simulink model "TestStructure"  (R2022b)
settings: Solver=FixedStepDiscrete  StartTime=0.0  StopTime=300  FixedStep=SampleTime  RelTol=1e-3
InitFcn:
  | SampleTime = 0.001;
  | ButtonValue=0;
  | load("BusConfig.mat");
model workspace (MAT data in the model file):
  Manual_Auto = 1
  Pattern = 1
  Pause_Start = 1
  Stop = 1
  Unlock_Lock = 1
undefined symbols (not defined in the file or in its folder): DiscIntNeverNeededParam
libraries: dspfdesign x4, dspstat3 x4
(part 1 of 3)
settings Model: SimulationMode=external  ExtModeEnableFloating=off  ExplicitPartitioning=on  Creator=My-Dell-PC  LastModifiedBy=Lenovo
settings SolverCC: ConcurrentTasks=on  PositivePriorityOrder=on
settings OptimizationCC: BlockReduction=off  OptimizeBlockIOStorage=off
settings DebuggingCC: TasksWithSamePriorityMsg=none
settings HardwareCC: ProdBitPerLong=64  ProdLongLongMode=on  ProdHWDeviceType=Intel->x86-64 (Linux 64)
settings RTWCC: Description=Simulink Real-Time  SystemTargetFile=slrealtime.tlc  TemplateMakefile=slrealtime_default_tmf  Toolchain=Simulink Real-Time Toolchain  BuildConfiguration=Faster Runs  CodeExecutionProfiling=on  TargetLang=C++
settings CodeAppCC: MaxIdLength=128

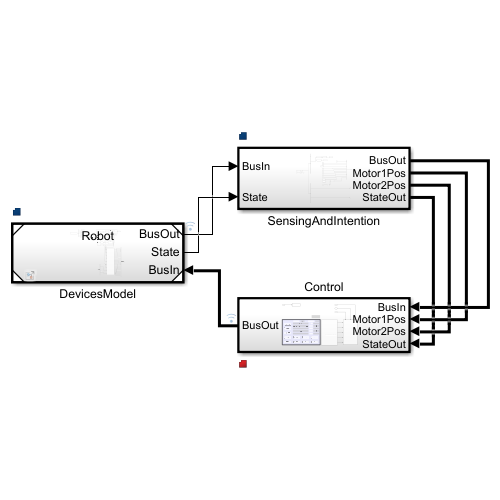
[thumbnail: Simulink's stored preview of the top-level diagram]
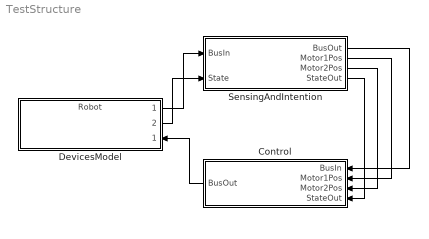
== system TestStructure ==
  Control : Subsystem  TreatAsAtomicUnit=on
  DevicesModel : ModelReference  ModelNameDialog=Robot.slx  SimulationMode=Normal  ModelReferenceVersion=1.102
      settings: PortSchema="{\"entries\":[{\"content\":{\"sides\":[{\"content\":{\"connectorIds\":[]},\"type\":\"ConnectorPlacement.EquallySpacedRectSide\",\"uuid\":\"7b8c9a1c-e183-4267-9de8-fd35f280369e\"},{\"content\":{\"connectorIds\":[\"Out1\",\"Out2\",\"In1\"],\"side\":\"RIGHT\"},\"type\":\"ConnectorPlacement.EquallySpacedRectSide\",\"uuid\":\"78ba3a26-fd01-47d1-83ec-a88a58443a5d\"},{\"content\":{\"connectorIds\":[],\"side\":\"TOP\"},\"type\":\"ConnectorPlacement.EquallySpacedRectSide\",\"uuid\":\"d4867a2f-46dd-4a62-ab42-9e8e97143c91\"}]},\"type\":\"ConnectorPlacement.EquallySpacedConnector\",\"uuid\":\"fb86ace7-67ae-423a-b56c-83b1d93efbca\"}],\"packageUris\":[\"http://schema.mathworks.com/mf0/Connector/R2020b\"],\"version\":\"1.0\"}"
  SensingAndIntention : Subsystem  TreatAsAtomicUnit=on
  wires:
  SensingAndIntention/1(BusOut) -> Control/1(BusIn)
  DevicesModel/1 -> SensingAndIntention/1(BusIn)
  Control/1(BusOut) -> DevicesModel/1
  SensingAndIntention/2(Motor1Pos) -> Control/2(Motor1Pos)
  SensingAndIntention/3(Motor2Pos) -> Control/3(Motor2Pos)
  DevicesModel/2 -> SensingAndIntention/2(State)
  SensingAndIntention/4(StateOut) -> Control/4(StateOut)

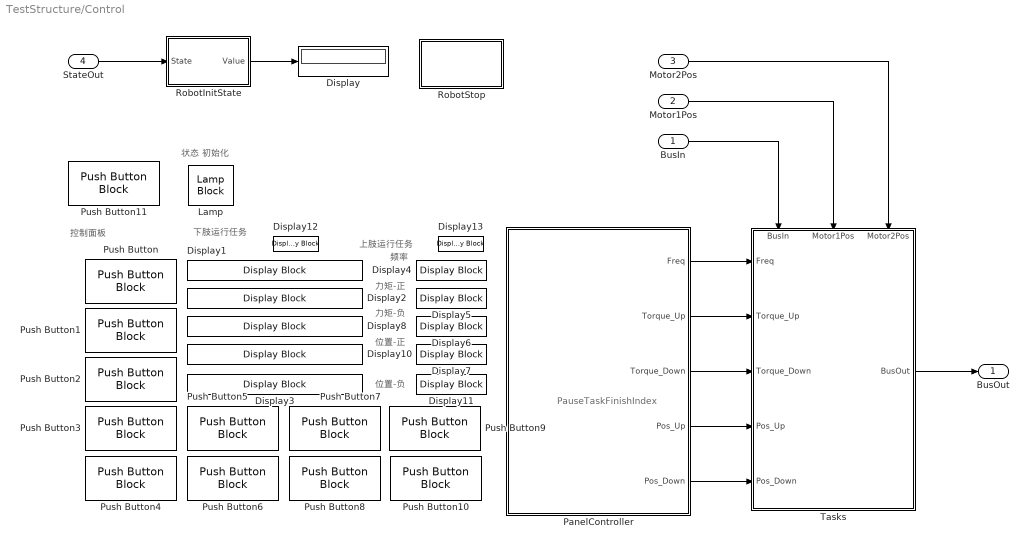
== system TestStructure/Control ==
  note: 状态 初始化
  note: PauseTaskFinishIndex
  note: 频率
  note: 控制面板
  note: 下肢运行任务
  note: 力矩-负
  note: 位置-负
  note: 位置-正
  note: 上肢运行任务
  note: 力矩-正
  BusIn : Inport  OutDataTypeStr=Bus: IntentionBus  BusOutputAsStruct=on
  Motor1Pos : Inport  Port=2
  Motor2Pos : Inport  Port=3
  StateOut : Inport  Port=4
  Display : Display
  Display{1..8,10..13} (12 alike) : DisplayBlock  LabelPosition=Hide  Transparency=1
  Lamp : LampBlock  LabelPosition=Hide
  PanelController : Subsystem  mask{LLFK_Freq_init=0.5, LLB_Freq_init=0.7, LLW_Freq_init=0.7, LLFK_Torque_Up_init=3, LLB_Torque_Up_init=9, LLW_Torque_Up_init=9, LLFK_Torque_Down_init=3, LLB_Torque_Down_init=9, LLW_Torque_Down_init=9, LLFK_Pos_Up_init=35, LLB_Pos_Up_init=80, LLW_Pos_Up_init=80, LLFK_Pos_Down_init=10, LLB_Pos_Down_init=120, LLW_Pos_Down_init=120}
      mask prompts: LLFK_Freq_init "LLFK_Freq_init (Hz)"; LLB_Freq_init "LLB_Freq_init (Hz)"; LLW_Freq_init "LLW_Freq_init (Hz)"; LLFK_Torque_Up_init "LLFK_Torque_Up_init (A)"; LLB_Torque_Up_init "LLB_Torque_Up_init (A)"; LLW_Torque_Up_init "LLW_Torque_Up_init (A)"; LLFK_Torque_Down_init "LLFK_Torque_Down_init (A)"; LLB_Torque_Down_init "LLB_Torque_Down_init (A)"; LLW_Torque_Down_init "LLW_Torque_Down_init (A)"; LLFK_Pos_Up_init "LLFK_Pos_Up_init (Degree)"; LLB_Pos_Up_init "LLB_Pos_Up_init (Degree)"; LLW_Pos_Up_init "LLW_Pos_Up_init (Degree)"; LLFK_Pos_Down_init "LLFK_Pos_Down_init (Degree)"; LLB_Pos_Down_init "LLB_Pos_Down_init (Degree)"; LLW_Pos_Down_init "LLW_Pos_Down_init (Degree)"
      mask DialogControl ParameterGroupVar Prompt: Freq_Init
      mask DialogControl Container3 Prompt: Torque_Up_Init
      mask DialogControl Container4 Prompt: Torque_Down_Init
      mask DialogControl Container5 Prompt: Pos_Up_init (Degree)
      mask DialogControl Container6 Prompt: Pos_Down_init (Degree)
  Push Button : PushButtonBlock  ButtonText=停止  Icon=Circle  IconColor=On  OffValue=0.000000
  Push Button1 : PushButtonBlock  ButtonText=启动/暂停  Icon=Circle  IconColor=On  OffValue=0.000000
  Push Button10 : PushButtonBlock  ButtonText=反方向-降  Icon=Circle  IconColor=On  OffValue=0.000000
  Push Button11 : PushButtonBlock  ButtonText=停止运行  Icon=Circle  IconColor=On  OffValue=0.000000
  Push Button2 : PushButtonBlock  ButtonText=模式  Icon=Circle  IconColor=On  OffValue=0.000000
  Push Button3 : PushButtonBlock  ButtonText=手动/自动  Icon=Circle  IconColor=On  OffValue=0.000000
  Push Button4 : PushButtonBlock  ButtonText=解锁/锁定  Icon=Circle  IconColor=On  OffValue=0.000000
  Push Button5 : PushButtonBlock  ButtonText=频率-升  Icon=Circle  IconColor=On  OffValue=0.000000
  Push Button6 : PushButtonBlock  ButtonText=频率-降  Icon=Circle  IconColor=On  OffValue=0.000000
  Push Button7 : PushButtonBlock  ButtonText=正方向-升  Icon=Circle  IconColor=On  OffValue=0.000000
  Push Button8 : PushButtonBlock  ButtonText=正方向-降  Icon=Circle  IconColor=On  OffValue=0.000000
  Push Button9 : PushButtonBlock  ButtonText=反方向-升  Icon=Circle  IconColor=On  OffValue=0.000000
  RobotInitState : Subsystem
  RobotStop : Subsystem
  Tasks : Subsystem
      settings: PortSchema="{\"entries\":[{\"content\":{\"sides\":[{\"content\":{\"connectorIds\":[\"In1\",\"In2\",\"In3\",\"In4\",\"In5\"]},\"type\":\"ConnectorPlacement.EquallySpacedRectSide\",\"uuid\":\"0ec11ac4-f889-444c-a7a1-b805f1cc982e\"},{\"content\":{\"connectorIds\":[\"Out1\"],\"side\":\"RIGHT\"},\"type\":\"ConnectorPlacement.EquallySpacedRectSide\",\"uuid\":\"b6409299-698f-49d2-9688-e152db4860ad\"},{\"content\":{\"connectorIds\":[\"In6\",\"In7\",\"In8\"],\"side\":\"TOP\"},\"type\":\"ConnectorPlacement.EquallySpacedRectSide\",\"uuid\":\"7591a67b-fad9-4669-8b21-584a47590ab5\"}]},\"type\":\"ConnectorPlacement.EquallySpacedConnector\",\"uuid\":\"b9f00c1f-80f2-4712-ac04-91dc0cbf24cb\"}],\"packageUris\":[\"http://schema.mathworks.com/mf0/Connector/R2020b\"],\"version\":\"1.0\"}"
  BusOut : Outport  OutDataTypeStr=Bus: ControlBus  BusOutputAsStruct=on
  wires:
  BusIn/1 -> Tasks/6(BusIn)
  PanelController/2(Torque_Up) -> Tasks/2(Torque_Up)
  PanelController/1(Freq) -> Tasks/1(Freq)
  PanelController/5(Pos_Down) -> Tasks/5(Pos_Down)
  PanelController/3(Torque_Down) -> Tasks/3(Torque_Down)
  PanelController/4(Pos_Up) -> Tasks/4(Pos_Up)
  Tasks/1(BusOut) -> BusOut/1
  Motor1Pos/1 -> Tasks/7(Motor1Pos)
  Motor2Pos/1 -> Tasks/8(Motor2Pos)
  StateOut/1 -> RobotInitState/1(State)
  RobotInitState/1(Value) -> Display/1

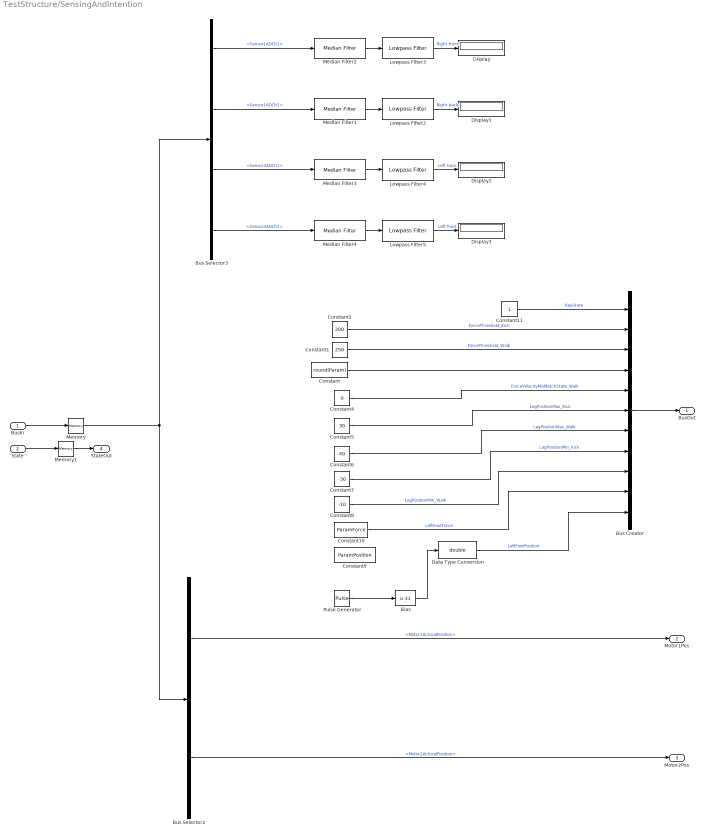
== system TestStructure/SensingAndIntention ==
  BusIn : Inport  OutDataTypeStr=Bus: SensingBus  BusOutputAsStruct=on
  State : Inport  Port=2
  Bias : Bias  Bias=-31  SaturateOnIntegerOverflow=off
  Bus Creator : BusCreator  Inputs=11  OutDataTypeStr=Bus: IntentionBus  NonVirtualBus=on
  Bus Selector2 : BusSelector  OutputSignals=Motor1ActuralPosition,Motor2ActuralPosition
  Bus Selector3 : BusSelector  OutputSignals=Sensor1ADCh1,Sensor1ADCh2,Sensor3ADCh1,Sensor3ADCh2
  Constant : Constant  Value=round(Param)  mask{Param=0.770}
  Constant1 : Constant  Value=250  OutDataTypeStr=double
  Constant10 : Constant  Value=ParamForce  OutDataTypeStr=double  mask{ParamForce=0.0}
  Constant11 : Constant  OutDataTypeStr=double
  Constant2 : Constant  Value=200  OutDataTypeStr=double
  Constant4 : Constant  Value=0  OutDataTypeStr=double
  Constant5 : Constant  Value=30  OutDataTypeStr=double
  Constant6 : Constant  Value=40  OutDataTypeStr=double
  Constant7 : Constant  Value=-30  OutDataTypeStr=double
  Constant8 : Constant  Value=-10  OutDataTypeStr=double
  Constant9 : Constant  Value=ParamPosition  OutDataTypeStr=double  mask{ParamPosition=1.860}
  Data Type Conversion : DataTypeConversion  OutDataTypeStr=double  SaturateOnIntegerOverflow=off  RndMeth=Floor
  Display{,1..3} (4 alike) : Display
  Lowpass Filter{2..5} (4 alike) : dspfdesign/Lowpass Filter  FilterType=IIR  DesignForMinimumOrder=off  FilterOrder=3  PassbandFrequency=3  StopbandFrequency=30  PassbandRipple=0.1  StopbandAttenuation=80  InheritSampleRate=off  SampleRate=1000  SimulateUsing=Code generation  roundingMode=Floor  coeffsDataTypeStr=fixdt(1,16)
  Median Filter{1..4} (4 alike) : dspstat3/Median Filter  WindowLength=80  SimulateUsing=Code generation
      settings: LibrarySourceBlock=|
      | dspfdesign/Median
      | Filter
  Memory : Memory
  Memory1 : Memory
  Pulse Generator : DiscretePulseGenerator  Amplitude=62  Period=T  PulseWidth=round(0.5*T)  PhaseDelay=round(0.5*T)  SampleTime=0.001  mask{T=2000.0}
  BusOut : Outport  OutDataTypeStr=Bus: IntentionBus  BusOutputAsStruct=on
  Motor1Pos : Outport  Port=2
  Motor2Pos : Outport  Port=3
  StateOut : Outport  Port=4
  wires:
  Bias/1 -> Data Type Conversion/1
  Constant1/1 -> Bus Creator/3  "ForceThreshold_Walk"
  Constant11/1 -> Bus Creator/1  "KeyState"
  Constant6/1 -> Bus Creator/7  "LegPositionMax_Walk"
  Data Type Conversion/1 -> Bus Creator/11  "LeftFootPosition"
  Constant2/1 -> Bus Creator/2  "ForceThreshold_Kick"
  Constant8/1 -> Bus Creator/9  "LegPositionMin_Walk"
  Constant7/1 -> Bus Creator/8  "LegPositionMin_Kick"
  Constant10/1 -> Bus Creator/10  "LeftFootForce"
  Constant4/1 -> Bus Creator/5  "ForceVelocityMisMatchState_Walk"
  Bus Creator/1 -> BusOut/1
  BusIn/1 -> Memory/1
  Constant5/1 -> Bus Creator/6  "LegPositionMax_Kick"
  Pulse Generator/1 -> Bias/1
  Bus Selector2/1 -> Motor1Pos/1  "<Motor1ActuralPosition>"
  Bus Selector2/2 -> Motor2Pos/1  "<Motor2ActuralPosition>"
  Memory/1 -> Bus Selector2/1, Bus Selector3/1
  Constant/1 -> Bus Creator/4
  Memory1/1 -> StateOut/1
  State/1 -> Memory1/1
  Median Filter1/1 -> Lowpass Filter2/1
  Median Filter2/1 -> Lowpass Filter3/1
  Bus Selector3/3 -> Median Filter3/1  "<Sensor3ADCh1>"
  Bus Selector3/1 -> Median Filter2/1  "<Sensor1ADCh1>"
  Median Filter4/1 -> Lowpass Filter5/1
  Bus Selector3/2 -> Median Filter1/1  "<Sensor1ADCh2>"
  Bus Selector3/4 -> Median Filter4/1  "<Sensor3ADCh2>"
  Median Filter3/1 -> Lowpass Filter4/1
  Lowpass Filter3/1 -> Display/1  "Right front"
  Lowpass Filter2/1 -> Display1/1  "Right back"
  Lowpass Filter4/1 -> Display2/1  "Left back"
  Lowpass Filter5/1 -> Display3/1  "Left front"

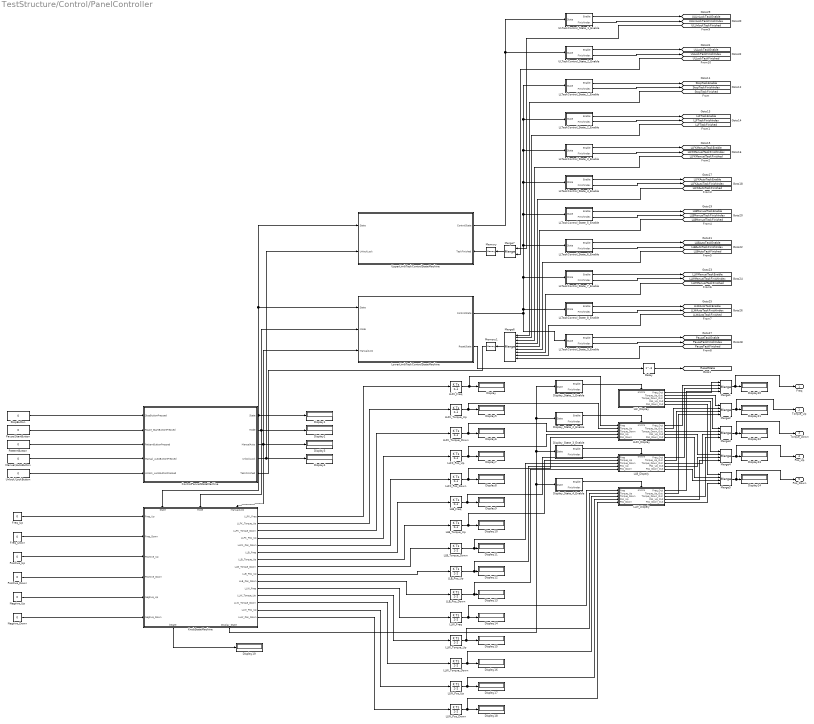
== system TestStructure/Control/PanelController ==
  ControlPannelStateMachine : Stateflow chart  TreatAsAtomicUnit=on
      settings: PortSchema="{\"entries\":[{\"content\":{\"sides\":[{\"content\":{\"connectorIds\":[\"In2\",\"In3\",\"In4\",\"In5\",\"In6\"]},\"type\":\"ConnectorPlacement.EquallySpacedRectSide\",\"uuid\":\"eab411cf-4b6a-48c6-b596-b66f8c420e7c\"},{\"content\":{\"connectorIds\":[\"Out1\",\"Out2\",\"Out3\",\"Out4\",\"In1\"],\"side\":\"RIGHT\"},\"type\":\"ConnectorPlacement.EquallySpacedRectSide\",\"uuid\":\"e0e09f46-7c1c-4140-8220-034119073277\"},{\"content\":{\"connectorIds\":[],\"side\":\"TOP\"},\"type\":\"ConnectorPlacement.EquallySpacedRectSide\",\"uuid\":\"ed6bf201-0ea3-4e7c-82a9-322f02ea728a\"}]},\"type\":\"ConnectorPlacement.EquallySpacedConnector\",\"uuid\":\"aa71b69e-402d-40b0-a3fd-c9400a9adadc\"}],\"packageUris\":[\"http://schema.mathworks.com/mf0/Connector/R2020b\"],\"version\":\"1.0\"}"
  Delay : Delay  DelayLength=3
  Display{,1..24} (25 alike) : Display
  Display_State_1_Enable : Subsystem  mask{TaskIndex=1}
  Display_State_2_Enable : Subsystem  mask{TaskIndex=2}
  Display_State_3_Enable : Subsystem  mask{TaskIndex=3}
  Display_State_4_Enable : Subsystem  mask{TaskIndex=4}
  Freq_Down : Constant  Value=0
  Freq_Up : Constant  Value=0
  KnobStateMachine : Stateflow chart  TreatAsAtomicUnit=on
      settings: PortSchema="{\"entries\":[{\"content\":{\"sides\":[{\"content\":{\"connectorIds\":[\"In1\",\"In2\",\"In3\",\"In4\",\"In5\",\"In6\"]},\"type\":\"ConnectorPlacement.EquallySpacedRectSide\",\"uuid\":\"78a56fe3-ceb0-42ee-90bc-aa39a12c9afb\"},{\"content\":{\"connectorIds\":[\"Out5\",\"Out3\",\"Out4\",\"Out6\",\"Out7\",\"Out8\",\"Out9\",\"Out10\",\"Out11\",\"Out12\",\"Out13\",\"Out14\",\"Out15\",\"Out16\",\"Out17\"],\"side\":\"RIGHT\"},\"type\":\"ConnectorPlacement.EquallySpacedRectSide\",\"uuid\":\"7553af84-a921-4f96-ace4-e42d4d568d32\"},{\"content\":{\"connectorIds\":[\"In7\",\"In8\",\"In9\"],\"side\":\"TOP\"},\"type\":\"ConnectorPlacement.EquallySpacedRectSide\",\"uuid\":\"299fd0e5-cc5b-4534-8b50-a134eaae2b47\"},{\"content\":{\"connectorIds\":[\"Out1\",\"Out2\"],\"side\":\"BOTTOM\"},\"type\":\"ConnectorPlacement.EquallySpacedRectSide\",\"uuid\":\"12262c62-fe5d-4494-9572-224afcc612c3\"}]},\"type\":\"ConnectorPlacement.EquallySpacedConnector\",\"uuid\":\"b0bd0f4e-3cef-462f-91f5-f8bdfcbb196f\"}],\"packageUris\":[\"http://schema.mathworks.com/mf0/Connector/R2020b\"],\"version\":\"1.0\"}"
  LLB_Dispaly : Subsystem
  LLB_Freq : DiscreteIntegrator  gainval=1000*0.1  InitialCondition=LLB_Freq_init  SampleTime=-1  LimitOutput=on  UpperSaturationLimit=2.5  LowerSaturationLimit=0.3  ICPrevOutput=DiscIntNeverNeededParam  ICPrevScaledInput=DiscIntNeverNeededParam
  LLB_Pos_Down : DiscreteIntegrator  gainval=1000*1  InitialCondition=LLB_Pos_Down_init  SampleTime=-1  LimitOutput=on  UpperSaturationLimit=140  LowerSaturationLimit=5  ICPrevOutput=DiscIntNeverNeededParam  ICPrevScaledInput=DiscIntNeverNeededParam
  LLB_Pos_Up : DiscreteIntegrator  gainval=1000*1  InitialCondition=LLB_Pos_Up_init  SampleTime=-1  LimitOutput=on  UpperSaturationLimit=100  LowerSaturationLimit=10  ICPrevOutput=DiscIntNeverNeededParam  ICPrevScaledInput=DiscIntNeverNeededParam
  LLB_Torque_Down : DiscreteIntegrator  gainval=1000*0.1  InitialCondition=LLB_Torque_Down_init  SampleTime=-1  LimitOutput=on  UpperSaturationLimit=10  LowerSaturationLimit=0  ICPrevOutput=DiscIntNeverNeededParam  ICPrevScaledInput=DiscIntNeverNeededParam
  LLB_Torque_Up : DiscreteIntegrator  gainval=1000*0.1  InitialCondition=LLB_Torque_Up_init  SampleTime=-1  LimitOutput=on  UpperSaturationLimit=10  LowerSaturationLimit=0  ICPrevOutput=DiscIntNeverNeededParam  ICPrevScaledInput=DiscIntNeverNeededParam
  LLFK_Display : Subsystem
  LLFK_Freq : DiscreteIntegrator  gainval=1000*0.1  InitialCondition=LLFK_Freq_init  SampleTime=-1  LimitOutput=on  UpperSaturationLimit=2.5  LowerSaturationLimit=0.3  ICPrevOutput=DiscIntNeverNeededParam  ICPrevScaledInput=DiscIntNeverNeededParam
  LLFK_Pos_Down : DiscreteIntegrator  gainval=1000*1  InitialCondition=LLFK_Pos_Down_init  SampleTime=-1  LimitOutput=on  UpperSaturationLimit=140  LowerSaturationLimit=5  ICPrevOutput=DiscIntNeverNeededParam  ICPrevScaledInput=DiscIntNeverNeededParam
  LLFK_Pos_Up : DiscreteIntegrator  gainval=1000*1  InitialCondition=LLFK_Pos_Up_init  SampleTime=-1  LimitOutput=on  UpperSaturationLimit=100  LowerSaturationLimit=10  ICPrevOutput=DiscIntNeverNeededParam  ICPrevScaledInput=DiscIntNeverNeededParam
  LLFK_Torque_Down : DiscreteIntegrator  gainval=1000*0.1  InitialCondition=LLFK_Torque_Down_init  SampleTime=-1  LimitOutput=on  UpperSaturationLimit=10  LowerSaturationLimit=0  ICPrevOutput=DiscIntNeverNeededParam  ICPrevScaledInput=DiscIntNeverNeededParam
  LLFK_Torque_Up : DiscreteIntegrator  gainval=1000*0.1  InitialCondition=LLFK_Torque_Up_init  SampleTime=-1  LimitOutput=on  UpperSaturationLimit=10  LowerSaturationLimit=0  ICPrevOutput=DiscIntNeverNeededParam  ICPrevScaledInput=DiscIntNeverNeededParam
  LLF_Display : Subsystem
  LLTaskControl_State_1_Enable : Subsystem  mask{TaskIndex=1}
  LLTaskControl_State_2_Enable : Subsystem  mask{TaskIndex=2}
  LLTaskControl_State_3_Enable : Subsystem  mask{TaskIndex=3}
  LLTaskControl_State_4_Enable : Subsystem  mask{TaskIndex=4}
  LLTaskControl_State_5_Enable : Subsystem  mask{TaskIndex=5}
  LLTaskControl_State_6_Enable : Subsystem  mask{TaskIndex=6}
  LLTaskControl_State_7_Enable : Subsystem  mask{TaskIndex=7}
  LLTaskControl_State_8_Enable : Subsystem  mask{TaskIndex=8}
  LLTaskControl_State_9_Enable : Subsystem  mask{TaskIndex=9}
  LLW_Dispaly : Subsystem
  LLW_Freq : DiscreteIntegrator  gainval=1000*0.1  InitialCondition=LLW_Freq_init  SampleTime=-1  LimitOutput=on  UpperSaturationLimit=2.5  LowerSaturationLimit=0.3  ICPrevOutput=DiscIntNeverNeededParam  ICPrevScaledInput=DiscIntNeverNeededParam
  LLW_Pos_Down : DiscreteIntegrator  gainval=1000*1  InitialCondition=LLW_Pos_Down_init  SampleTime=-1  LimitOutput=on  UpperSaturationLimit=140  LowerSaturationLimit=5  ICPrevOutput=DiscIntNeverNeededParam  ICPrevScaledInput=DiscIntNeverNeededParam
  LLW_Pos_Up : DiscreteIntegrator  gainval=1000*1  InitialCondition=LLW_Pos_Up_init  SampleTime=-1  LimitOutput=on  UpperSaturationLimit=100  LowerSaturationLimit=10  ICPrevOutput=DiscIntNeverNeededParam  ICPrevScaledInput=DiscIntNeverNeededParam
  LLW_Torque_Down : DiscreteIntegrator  gainval=1000*0.1  InitialCondition=LLW_Torque_Down_init  SampleTime=-1  LimitOutput=on  UpperSaturationLimit=10  LowerSaturationLimit=0  ICPrevOutput=DiscIntNeverNeededParam  ICPrevScaledInput=DiscIntNeverNeededParam
  LLW_Torque_Up : DiscreteIntegrator  gainval=1000*0.1  InitialCondition=LLW_Torque_Up_init  SampleTime=-1  LimitOutput=on  UpperSaturationLimit=10  LowerSaturationLimit=0  ICPrevOutput=DiscIntNeverNeededParam  ICPrevScaledInput=DiscIntNeverNeededParam
  LowerLimbTaskControlStateMachine : Stateflow chart  TreatAsAtomicUnit=on
  Manual/AutoButton : Constant  Value=0
  Memory : Memory
  Memory1 : Memory
  Merge{1..5} (5 alike) : Merge  Inputs=4
  Merge6 : Merge  Inputs=9
  Merge7 : Merge
  Negtive_Down : Constant  Value=0
  Negtive_Up : Constant  Value=0
  PatternButton : Constant  Value=0
  Pause/StartButton : Constant  Value=0
  Positive_Down : Constant  Value=0
  Positive_Up : Constant  Value=0
  StopButton : Constant  Value=0
  ULTaskControl_State_1_Enable : Subsystem  mask{TaskIndex=1}
  ULTaskControl_State_2_Enable : Subsystem  mask{TaskIndex=2}
  Unlock/LockButton : Constant  Value=0
  UpperLimbTaskControlStateMachine : Stateflow chart  TreatAsAtomicUnit=on
      settings: PortSchema="{\"entries\":[{\"content\":{\"sides\":[{\"content\":{\"connectorIds\":[\"In2\",\"In3\"]},\"type\":\"ConnectorPlacement.EquallySpacedRectSide\",\"uuid\":\"db13f0a7-324e-407f-8bcd-77b68e0b14b1\"},{\"content\":{\"connectorIds\":[\"Out1\",\"In1\"],\"side\":\"RIGHT\"},\"type\":\"ConnectorPlacement.EquallySpacedRectSide\",\"uuid\":\"09ee7819-fd71-4fe3-966c-1072161e5215\"},{\"content\":{\"connectorIds\":[],\"side\":\"TOP\"},\"type\":\"ConnectorPlacement.EquallySpacedRectSide\",\"uuid\":\"7aa19da4-9a31-402b-a0a8-4c1e281f7350\"}]},\"type\":\"ConnectorPlacement.EquallySpacedConnector\",\"uuid\":\"341b49cf-d13f-4e39-8c92-8137a597871d\"}],\"packageUris\":[\"http://schema.mathworks.com/mf0/Connector/R2020b\"],\"version\":\"1.0\"}"
  Freq : Outport
  Torque_Up : Outport  Port=2
  Torque_Down : Outport  Port=3
  Pos_Up : Outport  Port=4
  Pos_Down : Outport  Port=5
  tag scope: LLBAutoTaskEnable=global, LLBAutoTaskFinishIndex=global, LLBManualTaskEnable=global, LLBManualTaskFinishIndex=global, LLFKAutoTaskEnable=global, LLFKAutoTaskFinishIndex=global, LLFKManualTaskEnable=global, LLFKManualTaskFinishIndex=global, LLFTaskEnable=global, LLFTaskFinishIndex=global, LLWAutoTaskEnable=global, LLWAutoTaskFinishIndex=global, LLWManualTaskEnable=global, LLWManualTaskFinishIndex=global, PauseTaskEnable=global, PauseTaskFinishIndex=global, ResetState=global, StopTaskEnable=global, StopTaskFinishIndex=global, ULLockTaskEnable=global, ULLockTaskFinishIndex=global, ULUnLockTaskEnable=global, ULUnLockTaskFinishIndex=global
  wires:
  StopButton/1 -> ControlPannelStateMachine/2(StopButtonPressed)
  ControlPannelStateMachine/1(State) -> UpperLimbTaskControlStateMachine/2(State), LowerLimbTaskControlStateMachine/1(State), Display1/1, KnobStateMachine/7(State)
  Pause/StartButton/1 -> ControlPannelStateMachine/3(Pause_StartButtonPressed)
  PatternButton/1 -> ControlPannelStateMachine/4(PatternButtonPressed)
  Manual/AutoButton/1 -> ControlPannelStateMachine/5(Manual_AutoButtonPressed)
  ControlPannelStateMachine/2(Mode) -> KnobStateMachine/8(Mode), Display2/1, LowerLimbTaskControlStateMachine/2(Mode)
  ControlPannelStateMachine/3(ManualAuto) -> KnobStateMachine/9(ManualAuto), Display3/1, LowerLimbTaskControlStateMachine/3(ManualAuto)
  Unlock/LockButton/1 -> ControlPannelStateMachine/6(Unlock_LockButtonPressed)
  ControlPannelStateMachine/4(UnlockLock) -> Display4/1, UpperLimbTaskControlStateMachine/3(UnlockLock)
  LLFK_Freq/1 -> LLFK_Display/1(Freq), Display/1
  LLFK_Pos_Down/1 -> LLFK_Display/5(Pos_Down), Display8/1
  LLFK_Pos_Up/1 -> LLFK_Display/4(Pos_Up), Display7/1
  LLFK_Torque_Down/1 -> LLFK_Display/3(Torque_Down), Display6/1
  LLFK_Torque_Up/1 -> LLFK_Display/2(Torque_Up), Display5/1
  KnobStateMachine/5(LLFK_Freq) -> LLFK_Freq/1
  KnobStateMachine/3(LLFK_Torque_Up) -> LLFK_Torque_Up/1
  KnobStateMachine/4(LLFK_Torque_Down) -> LLFK_Torque_Down/1
  KnobStateMachine/6(LLFK_Pos_Up) -> LLFK_Pos_Up/1
  KnobStateMachine/7(LLFK_Pos_Down) -> LLFK_Pos_Down/1
  Freq_Up/1 -> KnobStateMachine/1(Freq_Up)
  Freq_Down/1 -> KnobStateMachine/2(Freq_Down)
  Positive_Up/1 -> KnobStateMachine/3(Positive_Up)
  Positive_Down/1 -> KnobStateMachine/4(Positive_Down)
  Negtive_Up/1 -> KnobStateMachine/5(Negtive_Up)
  Negtive_Down/1 -> KnobStateMachine/6(Negtive_Down)
  KnobStateMachine/9(LLB_Torque_Up) -> LLB_Torque_Up/1
  LLB_Pos_Up/1 -> LLB_Dispaly/4(Pos_Up), Display12/1
  KnobStateMachine/11(LLB_Pos_Up) -> LLB_Pos_Up/1
  LLB_Torque_Down/1 -> Display11/1, LLB_Dispaly/3(Torque_Down)
  LLB_Pos_Down/1 -> LLB_Dispaly/5(Pos_Down), Display13/1
  KnobStateMachine/10(LLB_Torque_Down) -> LLB_Torque_Down/1
  KnobStateMachine/12(LLB_Pos_Down) -> LLB_Pos_Down/1
  LLB_Freq/1 -> LLB_Dispaly/1(Freq), Display9/1
  LLB_Torque_Up/1 -> Display10/1, LLB_Dispaly/2(Torque_Up)
  KnobStateMachine/8(LLB_Freq) -> LLB_Freq/1
  KnobStateMachine/14(LLW_Torque_Up) -> LLW_Torque_Up/1
  LLW_Pos_Up/1 -> LLW_Dispaly/4(Pos_Up), Display17/1
  KnobStateMachine/16(LLW_Pos_Up) -> LLW_Pos_Up/1
  LLW_Torque_Down/1 -> LLW_Dispaly/3(Torque_Down), Display16/1
  KnobStateMachine/15(LLW_Torque_Down) -> LLW_Torque_Down/1
  KnobStateMachine/17(LLW_Pos_Down) -> LLW_Pos_Down/1
  LLW_Freq/1 -> LLW_Dispaly/1(Freq), Display14/1
  KnobStateMachine/13(LLW_Freq) -> LLW_Freq/1
  LLW_Torque_Up/1 -> LLW_Dispaly/2(Torque_Up), Display15/1
  LLW_Pos_Down/1 -> LLW_Dispaly/5(Pos_Down), Display18/1
  KnobStateMachine/1(kState) -> Display19/1
  Display_State_1_Enable/1(Enable) -> LLF_Display/Enable
  Display_State_2_Enable/1(Enable) -> LLFK_Display/Enable
  Display_State_3_Enable/1(Enable) -> LLB_Dispaly/Enable
  Display_State_4_Enable/1(Enable) -> LLW_Dispaly/Enable
  Merge1/1 -> Freq/1, Display20/1
  Merge2/1 -> Torque_Up/1, Display21/1
  Merge3/1 -> Torque_Down/1, Display22/1
  Merge4/1 -> Pos_Up/1, Display23/1
  Merge5/1 -> Pos_Down/1, Display24/1
  KnobStateMachine/2(Display_State) -> Display_State_1_Enable/1(State), Display_State_2_Enable/1(State), Display_State_3_Enable/1(State), Display_State_4_Enable/1(State)
  LLF_Display/1(Freq_Out) -> Merge1/1
  LLFK_Display/1(Freq_Out) -> Merge1/2
  LLB_Dispaly/1(Freq_Out) -> Merge1/3
  LLW_Dispaly/1(Freq_Out) -> Merge1/4
  LLF_Display/2(Torque_Up_Out) -> Merge2/1
  LLFK_Display/2(Torque_Up_Out) -> Merge2/2
  LLB_Dispaly/2(Torque_Up_Out) -> Merge2/3
  LLW_Dispaly/2(Torque_Up_Out) -> Merge2/4
  LLF_Display/3(Torque_Down_Out) -> Merge3/1
  LLFK_Display/3(Torque_Down_Out) -> Merge3/2
  LLB_Dispaly/3(Torque_Down_Out) -> Merge3/3
  LLW_Dispaly/3(Torque_Down_Out) -> Merge3/4
  LLF_Display/4(Pos_Up_Out) -> Merge4/1
  LLFK_Display/4(Pos_Up_Out) -> Merge4/2
  LLB_Dispaly/4(Pos_Up_Out) -> Merge4/3
  LLW_Dispaly/4(Pos_Up_Out) -> Merge4/4
  LLF_Display/5(Pos_Down_Out) -> Merge5/1
  LLFK_Display/5(Pos_Down_Out) -> Merge5/2
  LLB_Dispaly/5(Pos_Down_Out) -> Merge5/3
  LLW_Dispaly/5(Pos_Down_Out) -> Merge5/4
  [StopTaskFinished] -> Merge6/1
  LowerLimbTaskControlStateMachine/1(ControlState) -> LLTaskControl_State_1_Enable/1(State), LLTaskControl_State_2_Enable/1(State), LLTaskControl_State_3_Enable/1(State), LLTaskControl_State_4_Enable/1(State), LLTaskControl_State_5_Enable/1(State), LLTaskControl_State_6_Enable/1(State), LLTaskControl_State_7_Enable/1(State), LLTaskControl_State_8_Enable/1(State), LLTaskControl_State_9_Enable/1(State)
  Merge6/1 -> Memory1/1
  [LLFTaskFinished] -> Merge6/2
  [LLFKManualTaskFinished] -> Merge6/3
  [LLBManualTaskFinished] -> Merge6/5
  [LLWManualTaskFinished] -> Merge6/7
  [PauseTaskFinished] -> Merge6/9
  [LLFKAutoTaskFinished] -> Merge6/4
  [LLBAutoTaskFinished] -> Merge6/6
  [LLWAutoTaskFinished] -> Merge6/8
  Merge7/1 -> Memory/1
  [ULUnlockTaskFinished] -> Merge7/1
  [ULLockTaskFinished] -> Merge7/2
  UpperLimbTaskControlStateMachine/1(ControlState) -> ULTaskControl_State_2_Enable/1(State), ULTaskControl_State_1_Enable/1(State)
  LLTaskControl_State_8_Enable/1(Enable) -> [LLWAutoTaskEnable]
  LLTaskControl_State_5_Enable/2(FinishIndex) -> [LLBManualTaskFinishIndex]
  LLTaskControl_State_8_Enable/2(FinishIndex) -> [LLWAutoTaskFinishIndex]
  LLTaskControl_State_7_Enable/2(FinishIndex) -> [LLWManualTaskFinishIndex]
  LLTaskControl_State_1_Enable/2(FinishIndex) -> [StopTaskFinishIndex]
  LLTaskControl_State_3_Enable/1(Enable) -> [LLFKManualTaskEnable]
  ULTaskControl_State_2_Enable/1(Enable) -> [ULLockTaskEnable]
  LLTaskControl_State_4_Enable/1(Enable) -> [LLFKAutoTaskEnable]
  ULTaskControl_State_1_Enable/2(FinishIndex) -> [ULUnLockTaskFinishIndex]
  LLTaskControl_State_9_Enable/1(Enable) -> [PauseTaskEnable]
  LLTaskControl_State_9_Enable/2(FinishIndex) -> [PauseTaskFinishIndex]
  LLTaskControl_State_3_Enable/2(FinishIndex) -> [LLFKManualTaskFinishIndex]
  LLTaskControl_State_4_Enable/2(FinishIndex) -> [LLFKAutoTaskFinishIndex]
  LLTaskControl_State_5_Enable/1(Enable) -> [LLBManualTaskEnable]
  LLTaskControl_State_2_Enable/1(Enable) -> [LLFTaskEnable]
  LLTaskControl_State_2_Enable/2(FinishIndex) -> [LLFTaskFinishIndex]
  LLTaskControl_State_1_Enable/1(Enable) -> [StopTaskEnable]
  LLTaskControl_State_6_Enable/2(FinishIndex) -> [LLBAutoTaskFinishIndex]
  LLTaskControl_State_6_Enable/1(Enable) -> [LLBAutoTaskEnable]
  ULTaskControl_State_2_Enable/2(FinishIndex) -> [ULLockTaskFinishIndex]
  LLTaskControl_State_7_Enable/1(Enable) -> [LLWManualTaskEnable]
  ULTaskControl_State_1_Enable/1(Enable) -> [ULUnLockTaskEnable]
  Memory/1 -> UpperLimbTaskControlStateMachine/1(TaskFinished)
  Memory1/1 -> ControlPannelStateMachine/1(TaskFinished)
  Delay/1 -> [ResetState]
  LowerLimbTaskControlStateMachine/2(ResetState) -> Delay/1

== system TestStructure/Control/RobotInitState ==
  State : Inport
  Constant : Constant  Value=0
  Constant1 : Constant
  If : If  IfExpression=u1 == 5
  If Action Subsystem : Subsystem  TreatAsAtomicUnit=on
  If Action Subsystem1 : Subsystem  TreatAsAtomicUnit=on
  Merge1 : Merge
  Value : Outport
  wires:
  If Action Subsystem1/1(Out1) -> Merge1/2
  State/1 -> If/1
  If/1 -> If Action Subsystem/Action
  If Action Subsystem/1(Out1) -> Merge1/1
  Constant1/1 -> If Action Subsystem/1(In1)
  If/2 -> If Action Subsystem1/Action
  Constant/1 -> If Action Subsystem1/1(In1)
  Merge1/1 -> Value/1

== system TestStructure/Control/RobotStop ==
  Constant : Constant  Value=0
  Stop Simulation : Stop
  wires:
  Constant/1 -> Stop Simulation/1

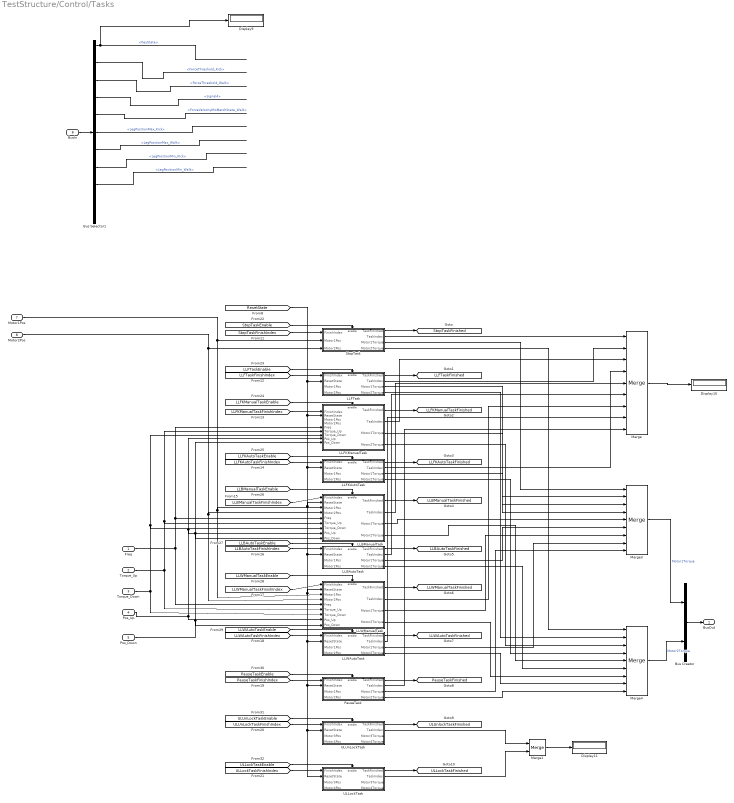
== system TestStructure/Control/Tasks ==
  Freq : Inport
  Torque_Up : Inport  Port=2
  Torque_Down : Inport  Port=3
  Pos_Up : Inport  Port=4
  Pos_Down : Inport  Port=5
  BusIn : Inport  Port=6  OutDataTypeStr=Bus: IntentionBus  BusOutputAsStruct=on
  Motor1Pos : Inport  Port=7
  Motor2Pos : Inport  Port=8
  Bus Creator : BusCreator  Inputs=2  OutDataTypeStr=Bus: ControlBus  NonVirtualBus=on
  Bus Selector1 : BusSelector  OutputSignals=KeyState,ForceThreshold_Kick,ForceThreshold_Walk,signal4,ForceVelocityMisMatchState_Walk,LegPositionMax_Kick,LegPositionMax_Walk,LegPositionMin_Kick,LegPositionMin_Walk,LeftFootForce,LeftFootPosition
  Display10 : Display
  Display11 : Display
  Display9 : Display
  LLBAutoTask : Subsystem
  LLBManualTask : Subsystem
  LLFKAutoTask : Subsystem
  LLFKManualTask : Subsystem
  LLFTask : Subsystem
  LLWAutoTask : Subsystem
  LLWManualTask : Subsystem
  Merge : Merge  Inputs=9
  Merge1 : Merge
  Merge3 : Merge  Inputs=9
  Merge4 : Merge  Inputs=9
  PauseTask : Subsystem
  StopTask : Subsystem
  ULLockTask : Subsystem
  ULUnLockTask : Subsystem
  BusOut : Outport  OutDataTypeStr=Bus: ControlBus  BusOutputAsStruct=on
  tag scope: LLBAutoTaskFinished=global, LLBManualTaskFinished=global, LLFKAutoTaskFinished=global, LLFKManualTaskFinished=global, LLFTaskFinished=global, LLWAutoTaskFinished=global, LLWManualTaskFinished=global, PauseTaskFinished=global, StopTaskFinished=global, ULLockTaskFinished=global, ULUnlockTaskFinished=global
  wires:
  ULLockTask/2(TaskIndex) -> Merge1/2
  LLFKAutoTask/2(TaskIndex) -> Merge/4
  LLFKManualTask/1(TaskFinished) -> [LLFKManualTaskFinished]
  [ULLockTaskFinishIndex] -> ULLockTask/1(FinishIndex)
  [ULUnLockTaskFinishIndex] -> ULUnLockTask/1(FinishIndex)
  Torque_Up/1 -> LLWManualTask/6(Torque_Up), LLBManualTask/6(Torque_Up), LLFKManualTask/6(Torque_Up)
  Pos_Down/1 -> LLBManualTask/9(Pos_Down), LLFKManualTask/9(Pos_Down), LLWManualTask/9(Pos_Down)
  ULUnLockTask/2(TaskIndex) -> Merge1/1
  LLWAutoTask/2(TaskIndex) -> Merge/8
  [LLBAutoTaskEnable] -> LLBAutoTask/Enable
  [LLBManualTaskFinishIndex] -> LLBManualTask/1(FinishIndex)
  [LLFKAutoTaskFinishIndex] -> LLFKAutoTask/1(FinishIndex)
  [LLFTaskEnable] -> LLFTask/Enable
  [ULLockTaskEnable] -> ULLockTask/Enable
  LLBManualTask/1(TaskFinished) -> [LLBManualTaskFinished]
  PauseTask/1(TaskFinished) -> [PauseTaskFinished]
  [LLBManualTaskEnable] -> LLBManualTask/Enable
  Merge/1 -> Display10/1
  Freq/1 -> LLWManualTask/5(Freq), LLBManualTask/5(Freq), LLFKManualTask/5(Freq)
  [LLFKManualTaskFinishIndex] -> LLFKManualTask/1(FinishIndex)
  PauseTask/2(TaskIndex) -> Merge/9
  Torque_Down/1 -> LLBManualTask/7(Torque_Down), LLFKManualTask/7(Torque_Down), LLWManualTask/7(Torque_Down)
  LLBManualTask/2(TaskIndex) -> Merge/5
  ULLockTask/1(TaskFinished) -> [ULLockTaskFinished]
  [StopTaskEnable] -> StopTask/Enable
  LLFTask/2(TaskIndex) -> Merge/2
  [PauseTaskFinishIndex] -> PauseTask/1(FinishIndex)
  LLWManualTask/1(TaskFinished) -> [LLWManualTaskFinished]
  Merge1/1 -> Display11/1
  LLFKAutoTask/1(TaskFinished) -> [LLFKAutoTaskFinished]
  [LLFKAutoTaskEnable] -> LLFKAutoTask/Enable
  [LLWManualTaskEnable] -> LLWManualTask/Enable
  Pos_Up/1 -> LLBManualTask/8(Pos_Up), LLFKManualTask/8(Pos_Up), LLWManualTask/8(Pos_Up)
  ULUnLockTask/1(TaskFinished) -> [ULUnlockTaskFinished]
  [LLWAutoTaskFinishIndex] -> LLWAutoTask/1(FinishIndex)
  [LLBAutoTaskFinishIndex] -> LLBAutoTask/1(FinishIndex)
  [LLWAutoTaskEnable] -> LLWAutoTask/Enable
  StopTask/1(TaskFinished) -> [StopTaskFinished]
  [LLFTaskFinishIndex] -> LLFTask/1(FinishIndex)
  LLFKManualTask/2(TaskIndex) -> Merge/3
  LLBAutoTask/2(TaskIndex) -> Merge/6
  LLFTask/1(TaskFinished) -> [LLFTaskFinished]
  [PauseTaskEnable] -> PauseTask/Enable
  [ULUnLockTaskEnable] -> ULUnLockTask/Enable
  [StopTaskFinishIndex] -> StopTask/1(FinishIndex)
  [LLFKManualTaskEnable] -> LLFKManualTask/Enable
  LLWManualTask/2(TaskIndex) -> Merge/7
  LLBAutoTask/1(TaskFinished) -> [LLBAutoTaskFinished]
  LLWAutoTask/1(TaskFinished) -> [LLWAutoTaskFinished]
  [LLWManualTaskFinishIndex] -> LLWManualTask/1(FinishIndex)
  StopTask/2(TaskIndex) -> Merge/1
  Merge4/1 -> Bus Creator/2  "Motor2Torque"
  Bus Creator/1 -> BusOut/1
  Merge3/1 -> Bus Creator/1  "Motor1Torque"
  Bus Selector1/8 -> ?  "<LegPositionMin_Kick>"
  Bus Selector1/3 -> ?  "<ForceThreshold_Walk>"
  Bus Selector1/7 -> ?  "<LegPositionMax_Walk>"
  Bus Selector1/5 -> ?  "<ForceVelocityMisMatchState_Walk>"
  Bus Selector1/9 -> ?  "<LegPositionMin_Walk>"
  Bus Selector1/2 -> ?  "<ForceThreshold_Kick>"
  Bus Selector1/4 -> ?  "<signal4>"
  Bus Selector1/1 -> Display9/1  "<KeyState>"
  Bus Selector1/6 -> ?  "<LegPositionMax_Kick>"
  BusIn/1 -> Bus Selector1/1
  StopTask/3(Motor1Torque) -> Merge3/1
  LLFTask/3(Motor1Torque) -> Merge3/2
  LLFKManualTask/3(Motor1Torque) -> Merge3/3
  LLFKAutoTask/3(Motor1Torque) -> Merge3/4
  LLBManualTask/3(Motor1Torque) -> Merge3/5
  LLBAutoTask/3(Motor1Torque) -> Merge3/6
  LLWManualTask/3(Motor1Torque) -> Merge3/7
  LLWAutoTask/3(Motor1Torque) -> Merge3/8
  PauseTask/3(Motor1Torque) -> Merge3/9
  StopTask/4(Motor2Torque) -> Merge4/1
  LLFTask/4(Motor2Torque) -> Merge4/2
  LLFKManualTask/4(Motor2Torque) -> Merge4/3
  LLFKAutoTask/4(Motor2Torque) -> Merge4/4
  LLBManualTask/4(Motor2Torque) -> Merge4/5
  LLBAutoTask/4(Motor2Torque) -> Merge4/6
  LLWManualTask/4(Motor2Torque) -> Merge4/7
  LLWAutoTask/4(Motor2Torque) -> Merge4/8
  PauseTask/4(Motor2Torque) -> Merge4/9
  Motor1Pos/1 -> LLWManualTask/3(Motor1Pos), LLBManualTask/3(Motor1Pos), StopTask/2(Motor1Pos)
  Motor2Pos/1 -> StopTask/3(Motor2Pos), LLWManualTask/4(Motor2Pos), LLBManualTask/4(Motor2Pos)
  [ResetState] -> LLFTask/2(ResetState), LLBManualTask/2(ResetState), ULLockTask/2(ResetState), ULUnLockTask/2(ResetState), PauseTask/2(ResetState), LLWAutoTask/2(ResetState), LLWManualTask/2(ResetState), LLBAutoTask/2(ResetState), LLFKAutoTask/2(ResetState), LLFKManualTask/2(ResetState)

== system TestStructure/Control/PanelController/Display_State_1_Enable ==
  State : Inport
  Subsystem : Subsystem
  Switch Case : SwitchCase  CaseConditions={TaskIndex}
  Enable : Outport
  FinishIndex : Outport  Port=2
  wires:
  Switch Case/2 -> Subsystem/2(Case Default)
  Switch Case/1 -> Subsystem/1(Case)
  Subsystem/2(FinishIndex) -> FinishIndex/1
  Subsystem/1(Enable) -> Enable/1
  State/1 -> Switch Case/1

== system TestStructure/Control/PanelController/Display_State_2_Enable ==
  State : Inport
  Subsystem : Subsystem
  Switch Case : SwitchCase  CaseConditions={TaskIndex}
  Enable : Outport
  FinishIndex : Outport  Port=2
  wires:
  Switch Case/2 -> Subsystem/2(Case Default)
  Switch Case/1 -> Subsystem/1(Case)
  Subsystem/2(FinishIndex) -> FinishIndex/1
  Subsystem/1(Enable) -> Enable/1
  State/1 -> Switch Case/1

== system TestStructure/Control/PanelController/Display_State_3_Enable ==
  State : Inport
  Subsystem : Subsystem
  Switch Case : SwitchCase  CaseConditions={TaskIndex}
  Enable : Outport
  FinishIndex : Outport  Port=2
  wires:
  Switch Case/2 -> Subsystem/2(Case Default)
  Switch Case/1 -> Subsystem/1(Case)
  Subsystem/2(FinishIndex) -> FinishIndex/1
  Subsystem/1(Enable) -> Enable/1
  State/1 -> Switch Case/1

== system TestStructure/Control/PanelController/Display_State_4_Enable ==
  State : Inport
  Subsystem : Subsystem
  Switch Case : SwitchCase  CaseConditions={TaskIndex}
  Enable : Outport
  FinishIndex : Outport  Port=2
  wires:
  Switch Case/2 -> Subsystem/2(Case Default)
  Switch Case/1 -> Subsystem/1(Case)
  Subsystem/2(FinishIndex) -> FinishIndex/1
  Subsystem/1(Enable) -> Enable/1
  State/1 -> Switch Case/1

== system TestStructure/Control/PanelController/LLB_Dispaly ==
  Freq : Inport
  Torque_Up : Inport  Port=2
  Torque_Down : Inport  Port=3
  Pos_Up : Inport  Port=4
  Pos_Down : Inport  Port=5
  Enable : EnablePort
  Freq_Out : Outport
  Torque_Up_Out : Outport  Port=2
  Torque_Down_Out : Outport  Port=3
  Pos_Up_Out : Outport  Port=4
  Pos_Down_Out : Outport  Port=5
  wires:
  Freq/1 -> Freq_Out/1
  Torque_Up/1 -> Torque_Up_Out/1
  Torque_Down/1 -> Torque_Down_Out/1
  Pos_Up/1 -> Pos_Up_Out/1
  Pos_Down/1 -> Pos_Down_Out/1

== system TestStructure/Control/PanelController/LLFK_Display ==
  Freq : Inport
  Torque_Up : Inport  Port=2
  Torque_Down : Inport  Port=3
  Pos_Up : Inport  Port=4
  Pos_Down : Inport  Port=5
  Enable : EnablePort
  Freq_Out : Outport
  Torque_Up_Out : Outport  Port=2
  Torque_Down_Out : Outport  Port=3
  Pos_Up_Out : Outport  Port=4
  Pos_Down_Out : Outport  Port=5
  wires:
  Freq/1 -> Freq_Out/1
  Torque_Up/1 -> Torque_Up_Out/1
  Torque_Down/1 -> Torque_Down_Out/1
  Pos_Up/1 -> Pos_Up_Out/1
  Pos_Down/1 -> Pos_Down_Out/1

== system TestStructure/Control/PanelController/LLF_Display ==
  Enable : EnablePort
  Constant{,1..4} (5 alike) : Constant  Value=0
  Freq_Out : Outport
  Torque_Up_Out : Outport  Port=2
  Torque_Down_Out : Outport  Port=3
  Pos_Up_Out : Outport  Port=4
  Pos_Down_Out : Outport  Port=5
  wires:
  Constant/1 -> Freq_Out/1
  Constant1/1 -> Torque_Up_Out/1
  Constant2/1 -> Torque_Down_Out/1
  Constant3/1 -> Pos_Up_Out/1
  Constant4/1 -> Pos_Down_Out/1

== system TestStructure/Control/PanelController/LLTaskControl_State_1_Enable ==
  State : Inport
  Subsystem : Subsystem
  Switch Case : SwitchCase  CaseConditions={TaskIndex}
  Enable : Outport
  FinishIndex : Outport  Port=2
  wires:
  Switch Case/2 -> Subsystem/2(Case Default)
  Switch Case/1 -> Subsystem/1(Case)
  Subsystem/2(FinishIndex) -> FinishIndex/1
  Subsystem/1(Enable) -> Enable/1
  State/1 -> Switch Case/1

== system TestStructure/Control/PanelController/LLTaskControl_State_2_Enable ==
  State : Inport
  Subsystem : Subsystem
  Switch Case : SwitchCase  CaseConditions={TaskIndex}
  Enable : Outport
  FinishIndex : Outport  Port=2
  wires:
  Switch Case/2 -> Subsystem/2(Case Default)
  Switch Case/1 -> Subsystem/1(Case)
  Subsystem/2(FinishIndex) -> FinishIndex/1
  Subsystem/1(Enable) -> Enable/1
  State/1 -> Switch Case/1

== system TestStructure/Control/PanelController/LLTaskControl_State_3_Enable ==
  State : Inport
  Subsystem : Subsystem
  Switch Case : SwitchCase  CaseConditions={TaskIndex}
  Enable : Outport
  FinishIndex : Outport  Port=2
  wires:
  Switch Case/2 -> Subsystem/2(Case Default)
  Switch Case/1 -> Subsystem/1(Case)
  Subsystem/2(FinishIndex) -> FinishIndex/1
  Subsystem/1(Enable) -> Enable/1
  State/1 -> Switch Case/1

== system TestStructure/Control/PanelController/LLTaskControl_State_4_Enable ==
  State : Inport
  Subsystem : Subsystem
  Switch Case : SwitchCase  CaseConditions={TaskIndex}
  Enable : Outport
  FinishIndex : Outport  Port=2
  wires:
  Switch Case/2 -> Subsystem/2(Case Default)
  Switch Case/1 -> Subsystem/1(Case)
  Subsystem/2(FinishIndex) -> FinishIndex/1
  Subsystem/1(Enable) -> Enable/1
  State/1 -> Switch Case/1

== system TestStructure/Control/PanelController/LLTaskControl_State_5_Enable ==
  State : Inport
  Subsystem : Subsystem
  Switch Case : SwitchCase  CaseConditions={TaskIndex}
  Enable : Outport
  FinishIndex : Outport  Port=2
  wires:
  Switch Case/2 -> Subsystem/2(Case Default)
  Switch Case/1 -> Subsystem/1(Case)
  Subsystem/2(FinishIndex) -> FinishIndex/1
  Subsystem/1(Enable) -> Enable/1
  State/1 -> Switch Case/1

== system TestStructure/Control/PanelController/LLTaskControl_State_6_Enable ==
  State : Inport
  Subsystem : Subsystem
  Switch Case : SwitchCase  CaseConditions={TaskIndex}
  Enable : Outport
  FinishIndex : Outport  Port=2
  wires:
  Switch Case/2 -> Subsystem/2(Case Default)
  Switch Case/1 -> Subsystem/1(Case)
  Subsystem/2(FinishIndex) -> FinishIndex/1
  Subsystem/1(Enable) -> Enable/1
  State/1 -> Switch Case/1

== system TestStructure/Control/PanelController/LLTaskControl_State_7_Enable ==
  State : Inport
  Subsystem : Subsystem
  Switch Case : SwitchCase  CaseConditions={TaskIndex}
  Enable : Outport
  FinishIndex : Outport  Port=2
  wires:
  Switch Case/2 -> Subsystem/2(Case Default)
  Switch Case/1 -> Subsystem/1(Case)
  Subsystem/2(FinishIndex) -> FinishIndex/1
  Subsystem/1(Enable) -> Enable/1
  State/1 -> Switch Case/1

== system TestStructure/Control/PanelController/LLTaskControl_State_8_Enable ==
  State : Inport
  Subsystem : Subsystem
  Switch Case : SwitchCase  CaseConditions={TaskIndex}
  Enable : Outport
  FinishIndex : Outport  Port=2
  wires:
  Switch Case/2 -> Subsystem/2(Case Default)
  Switch Case/1 -> Subsystem/1(Case)
  Subsystem/2(FinishIndex) -> FinishIndex/1
  Subsystem/1(Enable) -> Enable/1
  State/1 -> Switch Case/1

== system TestStructure/Control/PanelController/LLTaskControl_State_9_Enable ==
  State : Inport
  Subsystem : Subsystem
  Switch Case : SwitchCase  CaseConditions={TaskIndex}
  Enable : Outport
  FinishIndex : Outport  Port=2
  wires:
  Switch Case/2 -> Subsystem/2(Case Default)
  Switch Case/1 -> Subsystem/1(Case)
  Subsystem/2(FinishIndex) -> FinishIndex/1
  Subsystem/1(Enable) -> Enable/1
  State/1 -> Switch Case/1

== system TestStructure/Control/PanelController/LLW_Dispaly ==
  Freq : Inport
  Torque_Up : Inport  Port=2
  Torque_Down : Inport  Port=3
  Pos_Up : Inport  Port=4
  Pos_Down : Inport  Port=5
  Enable : EnablePort
  Freq_Out : Outport
  Torque_Up_Out : Outport  Port=2
  Torque_Down_Out : Outport  Port=3
  Pos_Up_Out : Outport  Port=4
  Pos_Down_Out : Outport  Port=5
  wires:
  Freq/1 -> Freq_Out/1
  Torque_Up/1 -> Torque_Up_Out/1
  Torque_Down/1 -> Torque_Down_Out/1
  Pos_Up/1 -> Pos_Up_Out/1
  Pos_Down/1 -> Pos_Down_Out/1

== system TestStructure/Control/PanelController/ULTaskControl_State_1_Enable ==
  State : Inport
  Subsystem : Subsystem
  Switch Case : SwitchCase  CaseConditions={TaskIndex}
  Enable : Outport
  FinishIndex : Outport  Port=2
  wires:
  Switch Case/2 -> Subsystem/2(Case Default)
  Switch Case/1 -> Subsystem/1(Case)
  Subsystem/2(FinishIndex) -> FinishIndex/1
  Subsystem/1(Enable) -> Enable/1
  State/1 -> Switch Case/1

== system TestStructure/Control/PanelController/ULTaskControl_State_2_Enable ==
  State : Inport
  Subsystem : Subsystem
  Switch Case : SwitchCase  CaseConditions={TaskIndex}
  Enable : Outport
  FinishIndex : Outport  Port=2
  wires:
  Switch Case/2 -> Subsystem/2(Case Default)
  Switch Case/1 -> Subsystem/1(Case)
  Subsystem/2(FinishIndex) -> FinishIndex/1
  Subsystem/1(Enable) -> Enable/1
  State/1 -> Switch Case/1

== system TestStructure/Control/RobotInitState/If Action Subsystem ==
  In1 : Inport
  Action Port : ActionPort  ActionPortLabel=if(u1 == 5)
  Out1 : Outport
  wires:
  In1/1 -> Out1/1

== system TestStructure/Control/RobotInitState/If Action Subsystem1 ==
  In1 : Inport
  Action Port : ActionPort  ActionPortLabel=else
  Out1 : Outport
  wires:
  In1/1 -> Out1/1

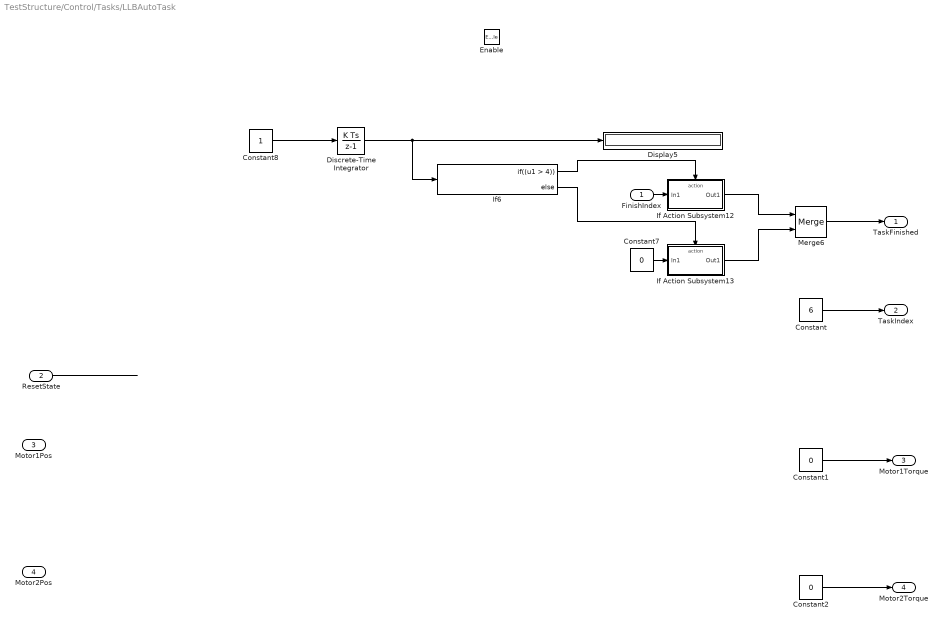
== system TestStructure/Control/Tasks/LLBAutoTask ==
  FinishIndex : Inport
  ResetState : Inport  Port=2
  Motor1Pos : Inport  Port=3
  Motor2Pos : Inport  Port=4
  Enable : EnablePort  StatesWhenEnabling=reset
  Constant : Constant  Value=6
  Constant1 : Constant  Value=0
  Constant2 : Constant  Value=0
  Constant7 : Constant  Value=0  OutDataTypeStr=double
  Constant8 : Constant
  Discrete-Time Integrator : DiscreteIntegrator  SampleTime=-1  ICPrevOutput=DiscIntNeverNeededParam  ICPrevScaledInput=DiscIntNeverNeededParam
  Display5 : Display
  If Action Subsystem12 : Subsystem  TreatAsAtomicUnit=on
  If Action Subsystem13 : Subsystem  TreatAsAtomicUnit=on
  If6 : If  IfExpression=(u1 > 4)
  Merge6 : Merge
  TaskFinished : Outport
  TaskIndex : Outport  Port=2
  Motor1Torque : Outport  Port=3
  Motor2Torque : Outport  Port=4
  wires:
  Merge6/1 -> TaskFinished/1
  If6/1 -> If Action Subsystem12/Action
  Constant8/1 -> Discrete-Time Integrator/1
  If6/2 -> If Action Subsystem13/Action
  Discrete-Time Integrator/1 -> If6/1, Display5/1
  If Action Subsystem13/1(Out1) -> Merge6/2
  FinishIndex/1 -> If Action Subsystem12/1(In1)
  If Action Subsystem12/1(Out1) -> Merge6/1
  Constant7/1 -> If Action Subsystem13/1(In1)
  Constant/1 -> TaskIndex/1
  Constant1/1 -> Motor1Torque/1
  Constant2/1 -> Motor2Torque/1
  ResetState/1 -> ?

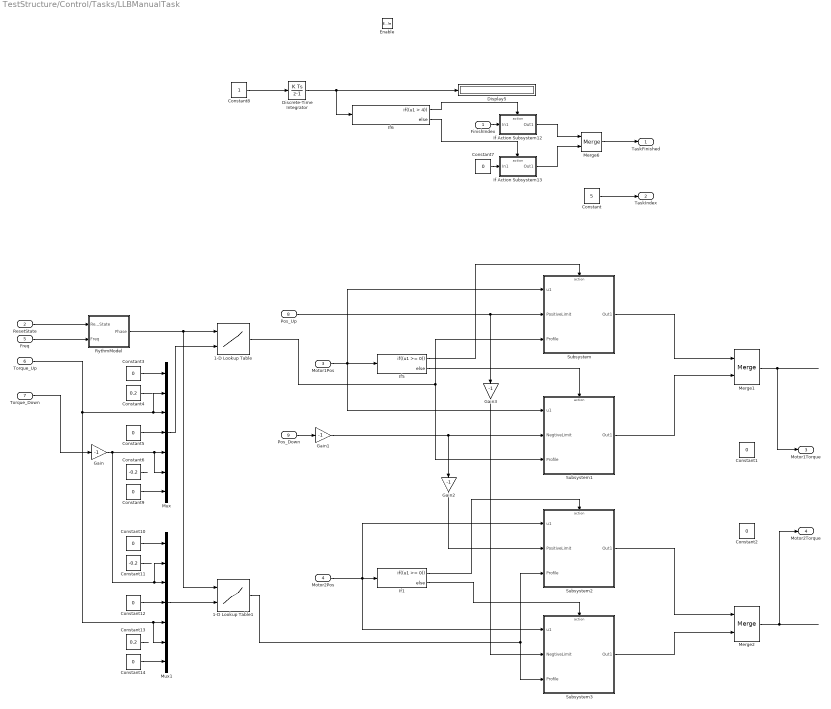
== system TestStructure/Control/Tasks/LLBManualTask ==
  FinishIndex : Inport
  ResetState : Inport  Port=2
  Motor1Pos : Inport  Port=3
  Motor2Pos : Inport  Port=4
  Freq : Inport  Port=5
  Torque_Up : Inport  Port=6
  Torque_Down : Inport  Port=7
  Pos_Up : Inport  Port=8
  Pos_Down : Inport  Port=9
  Enable : EnablePort  StatesWhenEnabling=reset
  1-D Lookup Table : Lookup_n-D  NumberOfTableDimensions=1  BreakpointsForDimension1=[0;0.2;0.35;0.5;0.65;0.85;1]  TableSource=Input port  Table=[0;0.2;3;0;-3;-0.2;0]  InternalRulePriority=Speed  RndMeth=Simplest
      settings: InputPortMap=u0,p221
  1-D Lookup Table1 : Lookup_n-D  NumberOfTableDimensions=1  BreakpointsForDimension1=[0;0.2;0.35;0.5;0.65;0.85;1]  TableSource=Input port  Table=[0;0.2;3;0;-3;-0.2;0]  InternalRulePriority=Speed  RndMeth=Simplest
      settings: InputPortMap=u0,p221
  Constant : Constant  Value=5
  Constant{1..3,5,9..10,12,14} (8 alike) : Constant  Value=0
  Constant11 : Constant  Value=-0.2
  Constant13 : Constant  Value=0.2
  Constant4 : Constant  Value=0.2
  Constant6 : Constant  Value=-0.2
  Constant7 : Constant  Value=0  OutDataTypeStr=double
  Constant8 : Constant
  Discrete-Time Integrator : DiscreteIntegrator  SampleTime=-1  ICPrevOutput=DiscIntNeverNeededParam  ICPrevScaledInput=DiscIntNeverNeededParam
  Display5 : Display
  Gain{,1..3} (4 alike) : Gain  Gain=-1
  If Action Subsystem12 : Subsystem  TreatAsAtomicUnit=on
  If Action Subsystem13 : Subsystem  TreatAsAtomicUnit=on
  If1 : If  IfExpression=(u1 >= 0)
  If5 : If  IfExpression=(u1 >= 0)
  If6 : If  IfExpression=(u1 > 4)
  Merge1 : Merge
  Merge2 : Merge
  Merge6 : Merge
  Mux : Mux  Inputs=7
  Mux1 : Mux  Inputs=7
  RythmModel : Subsystem
  Subsystem : Subsystem
  Subsystem1 : Subsystem
  Subsystem2 : Subsystem
  Subsystem3 : Subsystem
  TaskFinished : Outport
  TaskIndex : Outport  Port=2
  Motor1Torque : Outport  Port=3
  Motor2Torque : Outport  Port=4
  wires:
  Merge6/1 -> TaskFinished/1
  If6/1 -> If Action Subsystem12/Action
  Constant8/1 -> Discrete-Time Integrator/1
  If6/2 -> If Action Subsystem13/Action
  Discrete-Time Integrator/1 -> If6/1, Display5/1
  If Action Subsystem13/1(Out1) -> Merge6/2
  FinishIndex/1 -> If Action Subsystem12/1(In1)
  If Action Subsystem12/1(Out1) -> Merge6/1
  Constant7/1 -> If Action Subsystem13/1(In1)
  Constant/1 -> TaskIndex/1
  Gain1/1 -> Subsystem1/2(NegtiveLimit), Gain2/1
  Subsystem1/1(Out1) -> Merge1/2
  Pos_Down/1 -> Gain1/1
  Constant9/1 -> Mux/7
  Torque_Down/1 -> Gain/1
  Constant4/1 -> ?
  Constant13/1 -> ?
  Constant6/1 -> ?
  Freq/1 -> RythmModel/2(Freq)
  ResetState/1 -> RythmModel/1(ResetState)
  Mux/1 -> 1-D Lookup Table/2
  Subsystem2/1(Out1) -> Merge2/1
  Constant14/1 -> Mux1/7
  1-D Lookup Table/1 -> Subsystem1/3(Profile), Subsystem/3(Profile)
  Subsystem3/1(Out1) -> Merge2/2
  Pos_Up/1 -> Subsystem/2(PositiveLimit), Gain3/1
  If1/2 -> Subsystem3/Action
  Torque_Up/1 -> Mux1/6, Mux1/5, Mux/2, Mux/3
  Merge1/1 -> Motor1Torque/1
  RythmModel/1(Phase) -> 1-D Lookup Table1/1, 1-D Lookup Table/1
  Constant11/1 -> ?
  Constant10/1 -> Mux1/1
  Constant12/1 -> Mux1/4
  Constant5/1 -> Mux/4
  If1/1 -> Subsystem2/Action
  Constant3/1 -> Mux/1
  Motor2Pos/1 -> Subsystem3/1(u1), Subsystem2/1(u1), If1/1
  Motor1Pos/1 -> Subsystem1/1(u1), If5/1, Subsystem/1(u1)
  Mux1/1 -> 1-D Lookup Table1/2
  Gain/1 -> Mux1/2, Mux1/3, Mux/6, Mux/5
  If5/2 -> Subsystem1/Action
  1-D Lookup Table1/1 -> Subsystem2/3(Profile), Subsystem3/3(Profile)
  Gain2/1 -> Subsystem2/2(PositiveLimit)
  Merge2/1 -> Motor2Torque/1
  Subsystem/1(Out1) -> Merge1/1
  Gain3/1 -> Subsystem3/2(NegtiveLimit)
  If5/1 -> Subsystem/Action

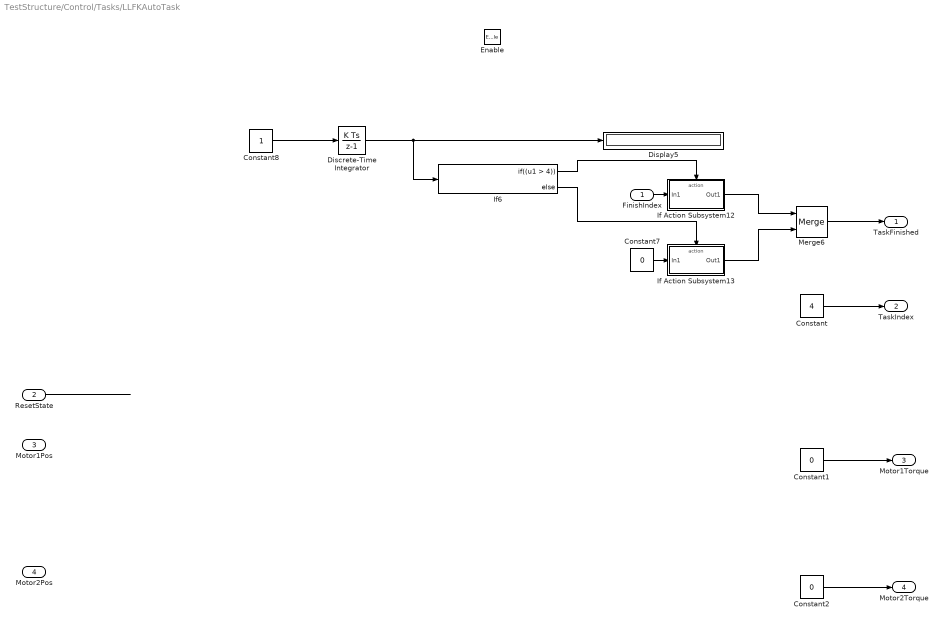
== system TestStructure/Control/Tasks/LLFKAutoTask ==
  FinishIndex : Inport
  ResetState : Inport  Port=2
  Motor1Pos : Inport  Port=3
  Motor2Pos : Inport  Port=4
  Enable : EnablePort  StatesWhenEnabling=reset
  Constant : Constant  Value=4
  Constant1 : Constant  Value=0
  Constant2 : Constant  Value=0
  Constant7 : Constant  Value=0  OutDataTypeStr=double
  Constant8 : Constant
  Discrete-Time Integrator : DiscreteIntegrator  SampleTime=-1  ICPrevOutput=DiscIntNeverNeededParam  ICPrevScaledInput=DiscIntNeverNeededParam
  Display5 : Display
  If Action Subsystem12 : Subsystem  TreatAsAtomicUnit=on
  If Action Subsystem13 : Subsystem  TreatAsAtomicUnit=on
  If6 : If  IfExpression=(u1 > 4)
  Merge6 : Merge
  TaskFinished : Outport
  TaskIndex : Outport  Port=2
  Motor1Torque : Outport  Port=3
  Motor2Torque : Outport  Port=4
  wires:
  Merge6/1 -> TaskFinished/1
  If6/1 -> If Action Subsystem12/Action
  Constant8/1 -> Discrete-Time Integrator/1
  If6/2 -> If Action Subsystem13/Action
  Discrete-Time Integrator/1 -> If6/1, Display5/1
  If Action Subsystem13/1(Out1) -> Merge6/2
  FinishIndex/1 -> If Action Subsystem12/1(In1)
  If Action Subsystem12/1(Out1) -> Merge6/1
  Constant7/1 -> If Action Subsystem13/1(In1)
  Constant/1 -> TaskIndex/1
  Constant1/1 -> Motor1Torque/1
  Constant2/1 -> Motor2Torque/1
  ResetState/1 -> ?

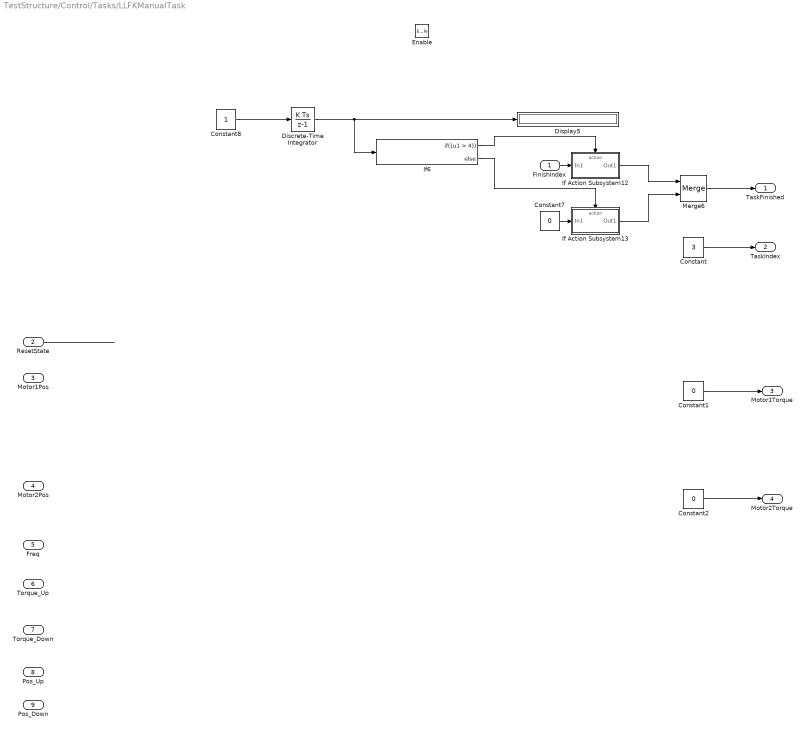
== system TestStructure/Control/Tasks/LLFKManualTask ==
  FinishIndex : Inport
  ResetState : Inport  Port=2
  Motor1Pos : Inport  Port=3
  Motor2Pos : Inport  Port=4
  Freq : Inport  Port=5
  Torque_Up : Inport  Port=6
  Torque_Down : Inport  Port=7
  Pos_Up : Inport  Port=8
  Pos_Down : Inport  Port=9
  Enable : EnablePort  StatesWhenEnabling=reset
  Constant : Constant  Value=3
  Constant1 : Constant  Value=0
  Constant2 : Constant  Value=0
  Constant7 : Constant  Value=0  OutDataTypeStr=double
  Constant8 : Constant
  Discrete-Time Integrator : DiscreteIntegrator  SampleTime=-1  ICPrevOutput=DiscIntNeverNeededParam  ICPrevScaledInput=DiscIntNeverNeededParam
  Display5 : Display
  If Action Subsystem12 : Subsystem  TreatAsAtomicUnit=on
  If Action Subsystem13 : Subsystem  TreatAsAtomicUnit=on
  If6 : If  IfExpression=(u1 > 4)
  Merge6 : Merge
  TaskFinished : Outport
  TaskIndex : Outport  Port=2
  Motor1Torque : Outport  Port=3
  Motor2Torque : Outport  Port=4
  wires:
  Merge6/1 -> TaskFinished/1
  If6/1 -> If Action Subsystem12/Action
  Constant8/1 -> Discrete-Time Integrator/1
  If6/2 -> If Action Subsystem13/Action
  Discrete-Time Integrator/1 -> If6/1, Display5/1
  If Action Subsystem13/1(Out1) -> Merge6/2
  FinishIndex/1 -> If Action Subsystem12/1(In1)
  If Action Subsystem12/1(Out1) -> Merge6/1
  Constant7/1 -> If Action Subsystem13/1(In1)
  Constant/1 -> TaskIndex/1
  Constant1/1 -> Motor1Torque/1
  Constant2/1 -> Motor2Torque/1
  ResetState/1 -> ?
